simulink model "Diagrama_distrito_personalizado"  (R2019a)
settings: Solver=VariableStepAuto  StartTime=0.0  StopTime=24  RelTol=1e-3
libraries: Libreria x14
settings Model: Creator=Usuario  LastModifiedBy=Usuario

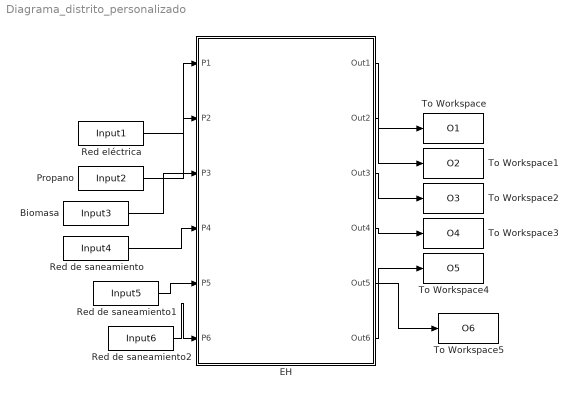
== system Diagrama_distrito_personalizado ==
  Biomasa : FromWorkspace  VariableName=Input3  SampleTime=0
  EH : Subsystem
  Propano : FromWorkspace  VariableName=Input2  SampleTime=0
  Red de saneamiento : FromWorkspace  VariableName=Input4  SampleTime=0
  Red de saneamiento1 : FromWorkspace  VariableName=Input5  SampleTime=0
  Red de saneamiento2 : FromWorkspace  VariableName=Input6  SampleTime=0
  Red eléctrica : FromWorkspace  VariableName=Input1  SampleTime=0
  To Workspace : ToWorkspace  VariableName=O1  SaveFormat=Timeseries  SampleTime=-1
  To Workspace1 : ToWorkspace  VariableName=O2  SaveFormat=Timeseries  SampleTime=-1
  To Workspace2 : ToWorkspace  VariableName=O3  SaveFormat=Timeseries  SampleTime=-1
  To Workspace3 : ToWorkspace  VariableName=O4  SaveFormat=Timeseries  SampleTime=-1
  To Workspace4 : ToWorkspace  VariableName=O5  SaveFormat=Timeseries  SampleTime=-1
  To Workspace5 : ToWorkspace  VariableName=O6  SaveFormat=Timeseries  SampleTime=-1
  wires:
  Red eléctrica/1 -> EH/1(P1)
  Propano/1 -> EH/2(P2)
  Biomasa/1 -> EH/3(P3)
  Red de saneamiento/1 -> EH/4(P4)
  EH/1(Out1) -> To Workspace/1
  EH/2(Out2) -> To Workspace1/1
  EH/3(Out3) -> To Workspace2/1
  EH/4(Out4) -> To Workspace3/1
  EH/6(Out6) -> To Workspace4/1
  Red de saneamiento1/1 -> EH/5(P5)
  Red de saneamiento2/1 -> EH/6(P6)
  EH/5(Out5) -> To Workspace5/1

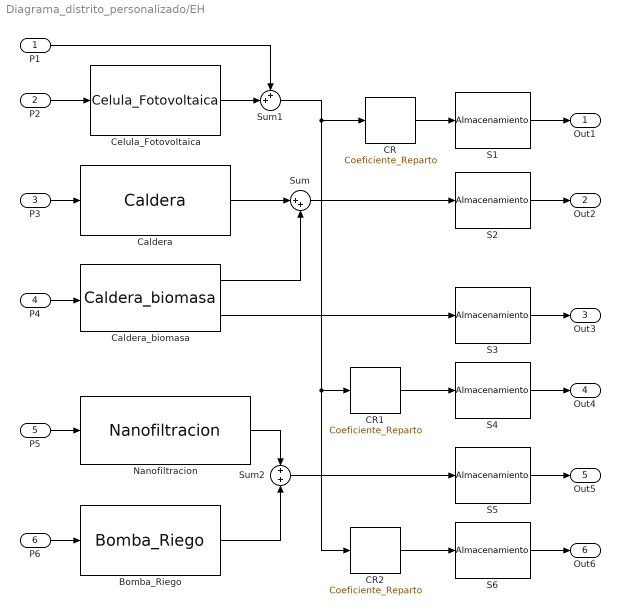
== system Diagrama_distrito_personalizado/EH ==
  P1 : Inport
  P2 : Inport  Port=2
  P3 : Inport  Port=3
  P4 : Inport  Port=4
  P5 : Inport  Port=5
  P6 : Inport  Port=6
  Bomba_Riego : Libreria/Bomba_Riego  efficiency=1  dispatch_factor=beta1  T_muestreo=T_muestreo  Max_in=150  Max_out=150  n_salida=[6]
      link override Funcion_coef_reparto: Tm=T_muestreo
  CR : Libreria/Coeficiente_Reparto  dispatch_factor=alfa1  Tm=T_muestreo  Max_out=inf  Max_in=inf  efficiency=1
  CR1 : Libreria/Coeficiente_Reparto  dispatch_factor=alfa2  Tm=T_muestreo  Max_out=inf  Max_in=inf  efficiency=1
  CR2 : Libreria/Coeficiente_Reparto  dispatch_factor=alfa3  Tm=T_muestreo  Max_out=inf  Max_in=inf  efficiency=1
  Caldera : Libreria/Caldera  efficiency=12  dispatch_factor=1  T_muestreo=T_muestreo  Min_in=0  Max_in=10  Max_out=120
  Caldera_biomasa : Libreria/Caldera_biomasa  efficiency=[12 7]  dispatch_factor=1  T_muestreo=T_muestreo  Max_in=10  Min_in=0  Max_out=[120 70]
  Celula_Fotovoltaica : Libreria/Celula_Fotovoltaica  efficiency=[3]  dispatch_factor=1  T_muestreo=T_muestreo  Max_in=1200  Max_out=2000
  Nanofiltracion : Libreria/Nanofiltracion  efficiency=0.95  dispatch_factor=beta2  T_muestreo=T_muestreo  Max_in=60  Max_out=60  n_salida=[4]
  S1 : Libreria/Almacenamiento  Up2=1  Low2=0  r_c=1  Up=1  Low=0  r_d=1  Up1=10  Low1=0  almacenamiento_inicial=0  cpa=1  almacenamiento_on=on
      link override In1: SampleTime=1
      link override Qch: VariableName=Qchp1
      link override Qdis: VariableName=Qdisp1
      link override almacenamiento: VariableName=almacen1
      link override discrepancias_almacenamiento: VariableName=discrepancias_almacenamiento1
      link override ef: VariableName=Ech1
      link override eff: VariableName=Edis1
  S2 : Libreria/Almacenamiento  Up2=3  Low2=0  r_c=1  Up=3  Low=0  r_d=1  Up1=15  Low1=0  almacenamiento_inicial=0  cpa=1  almacenamiento_on=on
      link override In1: SampleTime=1
      link override Qch: VariableName=Qchp2
      link override Qdis: VariableName=Qdisp2
      link override almacenamiento: VariableName=almacen2
      link override discrepancias_almacenamiento: VariableName=discrepancias_almacenamiento2
      link override ef: VariableName=Ech2
      link override eff: VariableName=Edis2
  S3 : Libreria/Almacenamiento  Up2=3  Low2=0  r_c=1  Up=3  Low=0  r_d=1  Up1=15  Low1=0  almacenamiento_inicial=0  cpa=1  almacenamiento_on=on
      link override In1: SampleTime=1
      link override Qch: VariableName=Qchp3
      link override Qdis: VariableName=Qdisp3
      link override almacenamiento: VariableName=almacen3
      link override discrepancias_almacenamiento: VariableName=discrepancias_almacenamiento3
      link override ef: VariableName=Ech3
      link override eff: VariableName=Edis3
  S4 : Libreria/Almacenamiento  Up2=1000  Low2=0  r_c=1  Up=1000  Low=0  r_d=1  Up1=1000  Low1=0  almacenamiento_inicial=0  cpa=1  almacenamiento_on=off
      link override In1: SampleTime=1
      link override Qch: VariableName=Qchp4
      link override Qdis: VariableName=Qdisp4
      link override almacenamiento: VariableName=almacen4
      link override discrepancias_almacenamiento: VariableName=discrepancias_almacenamiento4
      link override ef: VariableName=Ech4
      link override eff: VariableName=Edis4
  S5 : Libreria/Almacenamiento  Up2=100  Low2=0  r_c=1  Up=100  Low=0  r_d=1  Up1=500  Low1=0  almacenamiento_inicial=0  cpa=1  almacenamiento_on=on
      link override In1: SampleTime=1
      link override Qch: VariableName=Qchp5
      link override Qdis: VariableName=Qdisp5
      link override almacenamiento: VariableName=almacen5
      link override discrepancias_almacenamiento: VariableName=discrepancias_almacenamiento5
      link override ef: VariableName=Ech5
      link override eff: VariableName=Edis5
  S6 : Libreria/Almacenamiento  Up2=1000  Low2=0  r_c=1  Up=1000  Low=0  r_d=1  Up1=1000  Low1=0  almacenamiento_inicial=0  cpa=1  almacenamiento_on=off
      link override In1: SampleTime=1
      link override Qch: VariableName=Qchp6
      link override Qdis: VariableName=Qdisp6
      link override ef: VariableName=Ech6
      link override eff: VariableName=Edis6
  Sum : Sum  Inputs=|++
  Sum1 : Sum  Inputs=++|
  Sum2 : Sum
  Out1 : Outport
  Out2 : Outport  Port=2
  Out3 : Outport  Port=3
  Out4 : Outport  Port=4
  Out5 : Outport  Port=5
  Out6 : Outport  Port=6
  wires:
  Caldera/1 -> Sum/1
  CR/1 -> S1/1
  CR1/1 -> S4/1
  Sum/1 -> S2/1
  P1/1 -> Sum1/1
  Caldera_biomasa/2 -> S3/1
  Caldera_biomasa/1 -> Sum/2
  S4/1 -> Out4/1
  S3/1 -> Out3/1
  S2/1 -> Out2/1
  S1/1 -> Out1/1
  P2/1 -> Celula_Fotovoltaica/1
  Celula_Fotovoltaica/1 -> Sum1/2
  Sum1/1 -> CR2/1, CR1/1, CR/1
  P3/1 -> Caldera/1
  P4/1 -> Caldera_biomasa/1
  P5/1 -> Nanofiltracion/1
  S6/1 -> Out6/1
  Nanofiltracion/1 -> Sum2/1
  CR2/1 -> S6/1
  S5/1 -> Out5/1
  P6/1 -> Bomba_Riego/1
  Bomba_Riego/1 -> Sum2/2
  Sum2/1 -> S5/1
